simulink model "controller"  (R2022b)
settings: Solver=FixedStepAuto  StartTime=0.0  StopTime=10.0  FixedStep=1/100  RelTol=1e-3
undefined symbols (not defined in the file or in its folder): MAX_TORQUE, MAX_TORQUE_REVERSE
settings Model: Creator=DAUIN-Win10  LastModifiedBy=user
settings OptimizationCC: DefaultParameterBehavior=Inlined  EnhancedBackFolding=on  PassReuseOutputArgsAs=Individual arguments  ZeroExternalMemoryAtStartup=off  ZeroInternalMemoryAtStartup=off  OptimizeBlockOrder=speed  DifferentSizesBufferReuse=on  OptimizationCustomize=off  EfficientTunableParamExpr=on
settings DebuggingCC: ParameterTunabilityLossMsg=error  UnconnectedInputMsg=warning  UnconnectedOutputMsg=warning  UnconnectedLineMsg=warning
settings ModelReferenceCC: EnableRefExpFcnMdlSchedulingChecks=on
settings SFSimCC: MATLABDynamicMemAlloc=off
settings RTWCC: Description=Embedded Coder  SystemTargetFile=ert.tlc  TemplateMakefile=ert_default_tmf  DLArmComputeVersion=19.05
settings CodeAppCC: ForceParamTrailComments=on  IgnoreCustomStorageClasses=off  OperatorAnnotations=on  SimulinkDataObjDesc=on  SFDataObjDesc=on  InsertBlockDesc=on
settings ERTTargetCC: TargetLangStandard=C99 (ISO)  GenerateSampleERTMain=on  InlinedParameterPlacement=NonHierarchical  ERTCustomFileTemplate=example_file_process.tlc

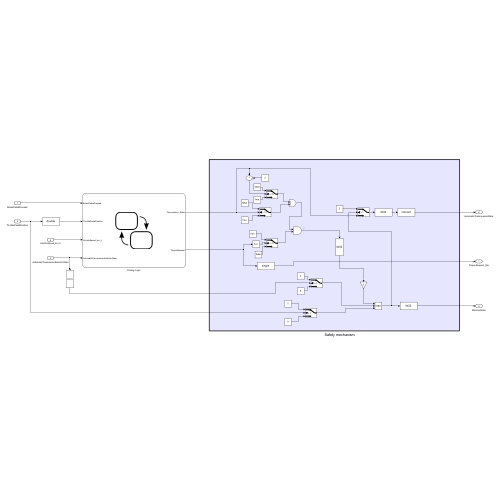
[thumbnail: Simulink's stored preview of the top-level diagram]
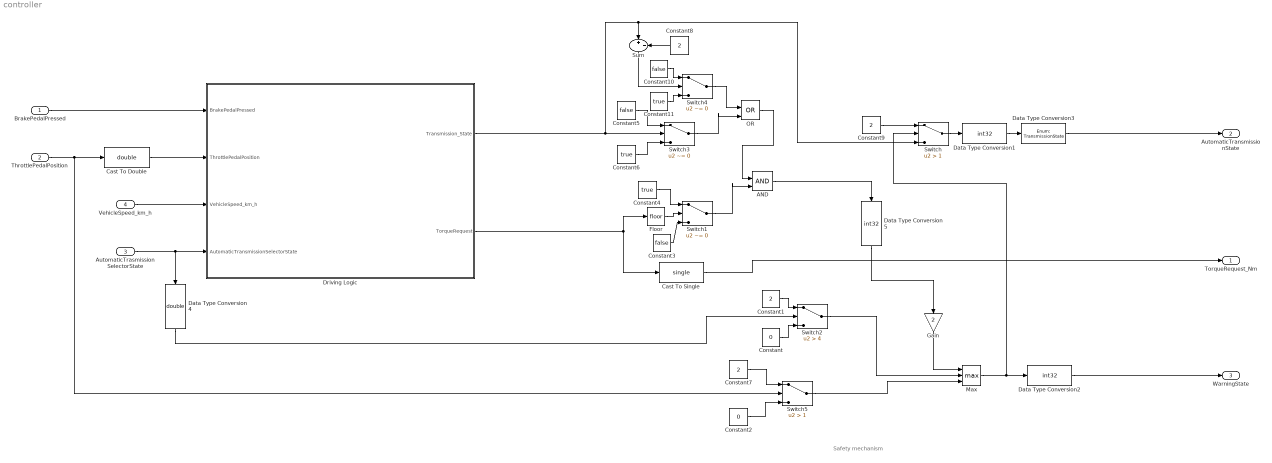
== system controller ==
  note: Safety mechanism
  BrakePedalPressed : Inport  OutDataTypeStr=boolean
  ThrottlePedalPosition : Inport  Port=2  OutDataTypeStr=single
  AutomaticTrasmissionSelectorState : Inport  Port=3  OutDataTypeStr=Enum: TransmissionState
  VehicleSpeed_km_h : Inport  Port=4  OutDataTypeStr=single  Unit=km/h
  AND : Logic  IconShape=distinctive  AllPortsSameDT=off  OutDataTypeStr=boolean
  Cast To Double : DataTypeConversion  OutDataTypeStr=double  SaturateOnIntegerOverflow=off  RndMeth=Floor
  Cast To Single : DataTypeConversion  OutDataTypeStr=single  SaturateOnIntegerOverflow=off  RndMeth=Floor
  Constant : Constant  Value=0
  Constant{1,7..9} (4 alike) : Constant  Value=2
  Constant10 : Constant  Value=false
  Constant11 : Constant  Value=true
  Constant2 : Constant  Value=0
  Constant3 : Constant  Value=false
  Constant4 : Constant  Value=true
  Constant5 : Constant  Value=false
  Constant6 : Constant  Value=true
  Data Type Conversion1 : DataTypeConversion  OutDataTypeStr=int32  SaturateOnIntegerOverflow=off  RndMeth=Floor  LockScale=on
  Data Type Conversion2 : DataTypeConversion  OutDataTypeStr=int32  SaturateOnIntegerOverflow=off  RndMeth=Floor
  Data Type Conversion3 : DataTypeConversion  OutDataTypeStr=Enum: TransmissionState  SaturateOnIntegerOverflow=off  RndMeth=Floor  LockScale=on
  Data Type Conversion4 : DataTypeConversion  OutDataTypeStr=double  SaturateOnIntegerOverflow=off  RndMeth=Floor
  Data Type Conversion5 : DataTypeConversion  OutDataTypeStr=int32  SaturateOnIntegerOverflow=off  RndMeth=Floor
  Driving Logic : Stateflow chart  TreatAsAtomicUnit=on
  Floor : Rounding
  Gain : Gain  Gain=2
  Max : MinMax  Function=max  Inputs=3
  OR : Logic  Operator=OR  IconShape=distinctive  AllPortsSameDT=off  OutDataTypeStr=boolean
  Sum : Sum  Inputs=|+-
  Switch : Switch  Criteria=u2 > Threshold  Threshold=1  SaturateOnIntegerOverflow=off  InputSameDT=off
  Switch1 : Switch  Criteria=u2 ~= 0  SaturateOnIntegerOverflow=off  InputSameDT=off
  Switch2 : Switch  Criteria=u2 > Threshold  Threshold=4  SaturateOnIntegerOverflow=off  InputSameDT=off
  Switch3 : Switch  Criteria=u2 ~= 0  SaturateOnIntegerOverflow=off  InputSameDT=off
  Switch4 : Switch  Criteria=u2 ~= 0  SaturateOnIntegerOverflow=off  InputSameDT=off
  Switch5 : Switch  Criteria=u2 > Threshold  Threshold=1  SaturateOnIntegerOverflow=off  InputSameDT=off
  TorqueRequest_Nm : Outport  OutDataTypeStr=single  Unit=N*m
  AutomaticTransmissionState : Outport  Port=2  OutDataTypeStr=Enum: TransmissionState
  WarningState : Outport  Port=3  OutDataTypeStr=int32
  wires:
  BrakePedalPressed/1 -> Driving Logic/1(BrakePedalPressed)
  AutomaticTrasmissionSelectorState/1 -> Driving Logic/4(AutomaticTransmissionSelectorState), Data Type Conversion4/1
  Driving Logic/2(TorqueRequest) -> Floor/1, Cast To Single/1
  Cast To Double/1 -> Driving Logic/2(ThrottlePedalPosition)
  Data Type Conversion3/1 -> AutomaticTransmissionState/1
  Data Type Conversion1/1 -> Data Type Conversion3/1
  Cast To Single/1 -> TorqueRequest_Nm/1
  Switch2/1 -> Max/2
  Data Type Conversion2/1 -> WarningState/1
  Constant1/1 -> Switch2/1
  VehicleSpeed_km_h/1 -> Driving Logic/3(VehicleSpeed_km_h)
  ThrottlePedalPosition/1 -> Switch5/2, Cast To Double/1
  Constant7/1 -> Switch5/1
  Switch5/1 -> Max/3
  Data Type Conversion4/1 -> Switch2/2
  Switch/1 -> Data Type Conversion1/1
  Max/1 -> Data Type Conversion2/1, Switch/2
  Driving Logic/1(Transmission_State) -> Switch/3, Sum/1, Switch3/2
  Constant9/1 -> Switch/1
  Constant/1 -> Switch2/3
  Constant2/1 -> Switch5/3
  Constant3/1 -> Switch1/3
  Constant4/1 -> Switch1/1
  Switch1/1 -> AND/2
  Constant5/1 -> Switch3/1
  Constant6/1 -> Switch3/3
  Constant8/1 -> Sum/2
  Constant10/1 -> Switch4/1
  Sum/1 -> Switch4/2
  Constant11/1 -> Switch4/3
  Switch4/1 -> OR/1
  Switch3/1 -> OR/2
  OR/1 -> AND/1
  AND/1 -> Data Type Conversion5/1
  Data Type Conversion5/1 -> Gain/1
  Gain/1 -> Max/1
  Floor/1 -> Switch1/2

== stateflow chart controller/Driving Logic ==
  state Park
    entry:
    TorqueRequest=0;
    Transmission_State=0;
  state Break
    entry:
    Transmission_State=4
    state Reg_Breaking_Region
      during:
      TorqueRequest=-MAX_TORQUE*(1-ThrottlePedalPosition*3);
    state Breaking_end
      entry:
      TorqueRequest=0;
    state Acceleration_Region
      during:
      TorqueRequest=MAX_TORQUE*3/2*(ThrottlePedalPosition - 1/3);
    Acceleration_Region -> Reg_Breaking_Region : [ ThrottlePedalPosition<=1/3]
    Reg_Breaking_Region -> Acceleration_Region [order 1] : [ThrottlePedalPosition>1/3]
    Reg_Breaking_Region -> Breaking_end [order 2] : [VehicleSpeed_km_h <=0.2]
    (default) -> Acceleration_Region
    Breaking_end -> Acceleration_Region : [ ThrottlePedalPosition >1/3]
  state Reverse
    entry:
    Transmission_State=1
    during:
    TorqueRequest = -ThrottlePedalPosition*MAX_TORQUE_REVERSE
  state Drive
    entry:
    Transmission_State=3
    during:
    TorqueRequest = ThrottlePedalPosition*MAX_TORQUE
  state Neutral
    entry:
    TorqueRequest=0;
    Transmission_State=2;
  (default) -> Park
  Neutral -> Park [order 3] : [abs(VehicleSpeed_km_h)<5 && BrakePedalPressed == 1 && AutomaticTransmissionSelectorState==0]
  Park -> Neutral : [BrakePedalPressed == 1 && AutomaticTransmissionSelectorState ~= 0]
  Break -> Drive : [AutomaticTransmissionSelectorState~=4]
  Neutral -> Reverse [order 1] : [VehicleSpeed_km_h < 5 && BrakePedalPressed == 1 && AutomaticTransmissionSelectorState==1]
  Drive -> Neutral [order 1] : [AutomaticTransmissionSelectorState<3]
  Drive -> Break [order 2] : [ThrottlePedalPosition > 1/3 && AutomaticTransmissionSelectorState==4]
  Neutral -> Drive [order 2] : [VehicleSpeed_km_h > -5 && BrakePedalPressed == 1 && AutomaticTransmissionSelectorState>2]
  Reverse -> Neutral : [AutomaticTransmissionSelectorState~=1]
  data: BrakePedalPressed input; ThrottlePedalPosition input; VehicleSpeed_km_h input; Transmission_State output; TorqueRequest output double; AutomaticTransmissionSelectorState input; MAX_TORQUE_REVERSE parameter; MAX_TORQUE parameter
